simulink model "A312_kynematics"  (R2022b)
settings: Solver=VariableStepAuto  StartTime=0.0  StopTime=1000  RelTol=1e-14  AbsTol=1e-15
undefined symbols (not defined in the file or in its folder): E0, gainx, gainy, gainz, Ix, Iy, Iz, w0
settings Model: Creator=virgi  LastModifiedBy=virgi

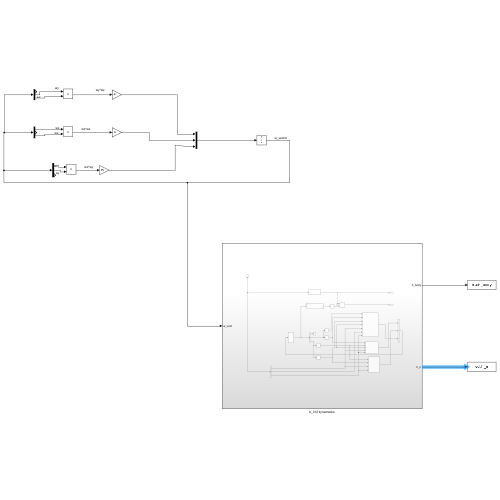
[thumbnail: Simulink's stored preview of the top-level diagram]
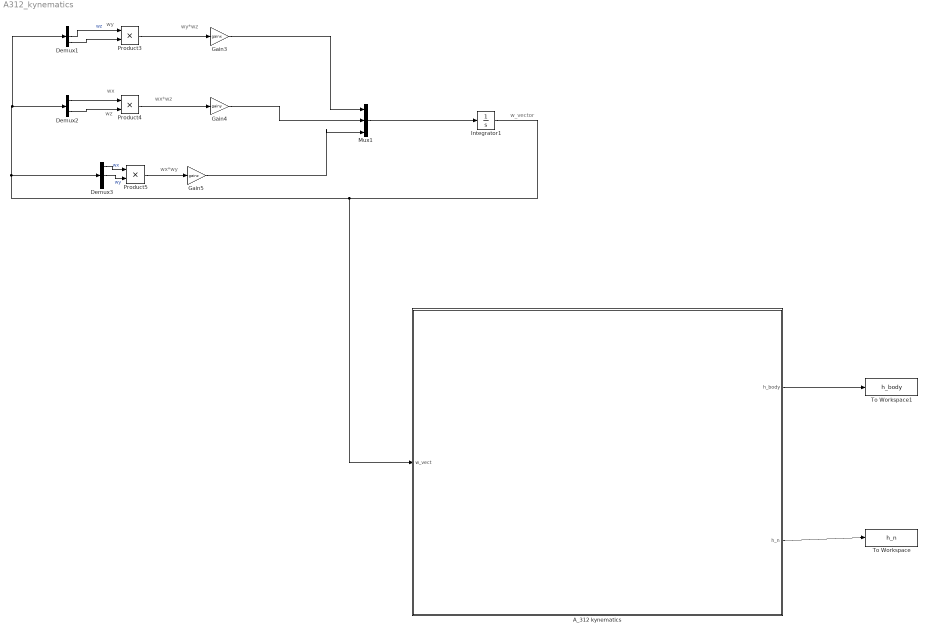
== system A312_kynematics ==
  note: w_vector
  note: wy
  note: wz
  note: wx*wy
  note: wy*wz
  note: wx*wz
  note: wx
  "A_312 kynematics " : Subsystem
  Demux1 : Demux  Outputs=3
  Demux2 : Demux  Outputs=3
  Demux3 : Demux  Outputs=3
  Gain3 : Gain  Gain=gainx
  Gain4 : Gain  Gain=gainy
  Gain5 : Gain  Gain=gainz
  Integrator1 : Integrator  InitialCondition=w0
  Mux1 : Mux  Inputs=3
  Product3 : Product
  Product4 : Product
  Product5 : Product
  To Workspace : ToWorkspace  VariableName=h_n  SampleTime=-1
  To Workspace1 : ToWorkspace  VariableName=h_body  SampleTime=-1
  wires:
  Demux3/2 -> Product5/2  "wy"
  Gain5/1 -> Mux1/3
  Demux2/3 -> Product4/2
  Demux3/1 -> Product5/1  "wx"
  Demux1/2 -> Product3/1  "wz"
  Demux1/3 -> Product3/2
  Integrator1/1 -> "A_312 kynematics "/1(w_vect), Demux1/1, Demux2/1, Demux3/1
  Demux2/1 -> Product4/1
  Gain4/1 -> Mux1/2
  Gain3/1 -> Mux1/1
  Product4/1 -> Gain4/1
  Product3/1 -> Gain3/1
  Product5/1 -> Gain5/1
  Mux1/1 -> Integrator1/1
  "A_312 kynematics "/1(h_body) -> To Workspace1/1
  "A_312 kynematics "/2(h_n) -> To Workspace/1

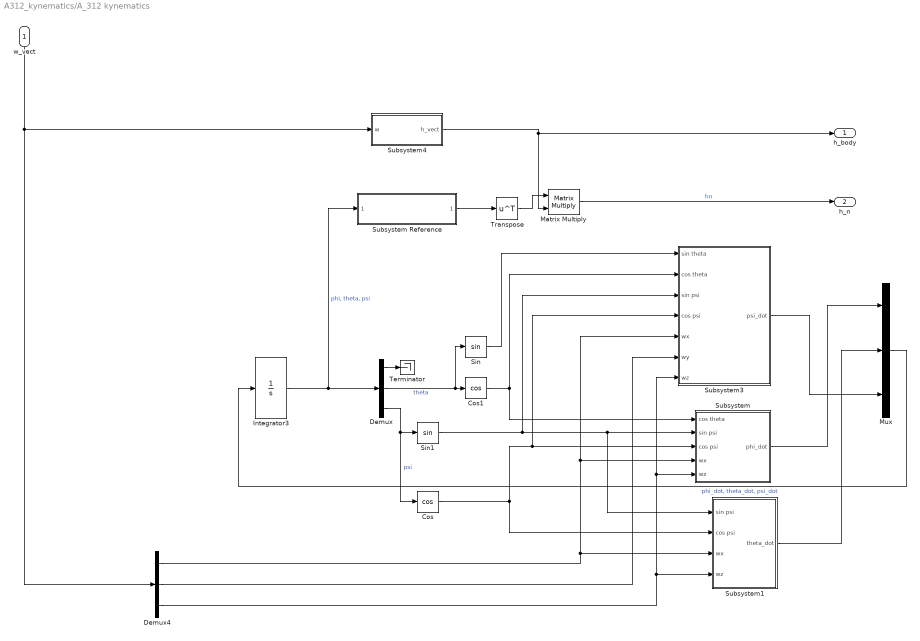
== system A312_kynematics/A_312 kynematics  ==
  w_vect : Inport
  Cos : Trigonometry  Operator=cos
  Cos1 : Trigonometry  Operator=cos
  Demux : Demux  Outputs=3
  Demux4 : Demux  Outputs=3
  Integrator3 : Integrator  InitialCondition=E0  WrapState=on
  Matrix Multiply : Product  Multiplication=Matrix(*)
  Mux : Mux  Inputs=3
  Sin : Trigonometry
  Sin1 : Trigonometry
  Subsystem : Subsystem
  Subsystem Reference : Subsystem  ReferencedSubsystem=A312
  Subsystem1 : Subsystem
  Subsystem3 : Subsystem
  Subsystem4 : Subsystem
  Terminator : Terminator
  Transpose : Math  Operator=transpose
  h_body : Outport
  h_n : Outport  Port=2
  wires:
  Demux/2 -> Sin/1, Cos1/1  "theta"
  Demux/3 -> Cos/1, Sin1/1  "psi"
  Demux4/1 -> Subsystem/4(wx), Subsystem3/5(wx), Subsystem1/3(wx)
  Sin1/1 -> Subsystem/2(sin psi), Subsystem1/1(sin psi), Subsystem3/3(sin psi)
  Subsystem4/1(h_vect) -> h_body/1, Matrix Multiply/2
  Matrix Multiply/1 -> h_n/1  "hn"
  Subsystem/1(phi_dot) -> Mux/1
  Integrator3/1 -> Subsystem Reference/1, Demux/1  "phi, theta, psi"
  Transpose/1 -> Matrix Multiply/1
  Subsystem3/1(psi_dot) -> Mux/3
  Demux4/3 -> Subsystem/5(wz), Subsystem3/7(wz), Subsystem1/4(wz)
  Cos1/1 -> Subsystem3/2(cos theta), Subsystem/1(cos theta)
  Cos/1 -> Subsystem3/4(cos psi), Subsystem/3(cos psi), Subsystem1/2(cos psi)
  Subsystem1/1(theta_dot) -> Mux/2
  Demux/1 -> Terminator/1
  Subsystem Reference/1 -> Transpose/1
  Mux/1 -> Integrator3/1  "phi_dot, theta_dot, psi_dot"
  Demux4/2 -> Subsystem3/6(wy)
  Sin/1 -> Subsystem3/1(sin theta)
  w_vect/1 -> Subsystem4/1(w), Demux4/1

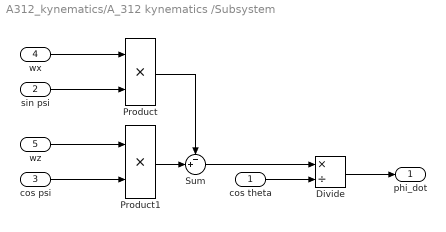
== system A312_kynematics/A_312 kynematics /Subsystem ==
  cos theta : Inport
  sin psi : Inport  Port=2
  cos psi : Inport  Port=3
  wx : Inport  Port=4
  wz : Inport  Port=5
  Divide : Product  Inputs=*/
  Product : Product
  Product1 : Product
  Sum : Sum  Inputs=-+|
  phi_dot : Outport
  wires:
  sin psi/1 -> Product/2
  wx/1 -> Product/1
  Product1/1 -> Sum/2
  cos theta/1 -> Divide/2
  Product/1 -> Sum/1
  cos psi/1 -> Product1/2
  Sum/1 -> Divide/1
  wz/1 -> Product1/1
  Divide/1 -> phi_dot/1

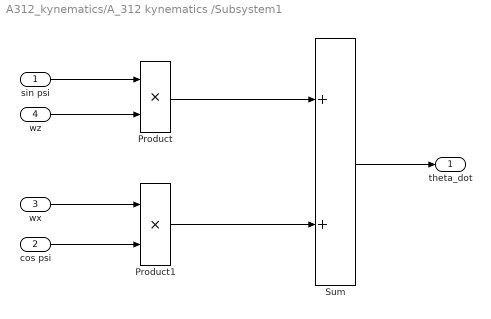
== system A312_kynematics/A_312 kynematics /Subsystem1 ==
  sin psi : Inport
  cos psi : Inport  Port=2
  wx : Inport  Port=3
  wz : Inport  Port=4
  Product : Product
  Product1 : Product
  Sum : Sum
  theta_dot : Outport
  wires:
  Product/1 -> Sum/1
  Product1/1 -> Sum/2
  cos psi/1 -> Product1/2
  wx/1 -> Product1/1
  wz/1 -> Product/2
  sin psi/1 -> Product/1
  Sum/1 -> theta_dot/1

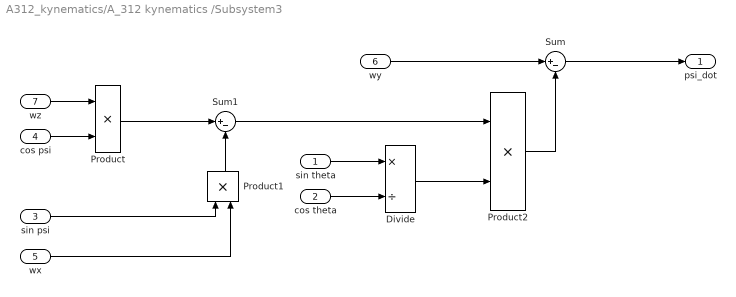
== system A312_kynematics/A_312 kynematics /Subsystem3 ==
  sin theta : Inport
  cos theta : Inport  Port=2
  sin psi : Inport  Port=3
  cos psi : Inport  Port=4
  wx : Inport  Port=5
  wy : Inport  Port=6
  wz : Inport  Port=7
  Divide : Product  Inputs=*/
  Product : Product
  Product1 : Product
  Product2 : Product
  Sum : Sum  Inputs=|+-
  Sum1 : Sum  Inputs=|+-
  psi_dot : Outport
  wires:
  wy/1 -> Sum/1
  Product1/1 -> Sum1/2
  wz/1 -> Product/1
  cos psi/1 -> Product/2
  Product/1 -> Sum1/1
  sin psi/1 -> Product1/1
  wx/1 -> Product1/2
  Sum1/1 -> Product2/1
  sin theta/1 -> Divide/1
  cos theta/1 -> Divide/2
  Divide/1 -> Product2/2
  Product2/1 -> Sum/2
  Sum/1 -> psi_dot/1

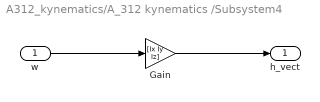
== system A312_kynematics/A_312 kynematics /Subsystem4 ==
  w : Inport
  Gain : Gain  Gain=[Ix Iy Iz]
  h_vect : Outport
  wires:
  w/1 -> Gain/1
  Gain/1 -> h_vect/1
